simulink model "Power_MIL"  (R2024b)
settings: Solver=FixedStepAuto  StartTime=0.0  StopTime=50.0  FixedStep=0.01  RelTol=1e-3
undefined symbols (not defined in the file or in its folder): dcVoltage, Np, Ns, RegulatorLogicControl_12, RegulatorLogicControl_3, RegulatorLogicControl_5, sensor
libraries: nesl_utility x24, fl_lib x21, ee_lib x5, batt_lib x1, autolibdatasheetbattery x1, autolibdcdc x1
(part 2 of 2)

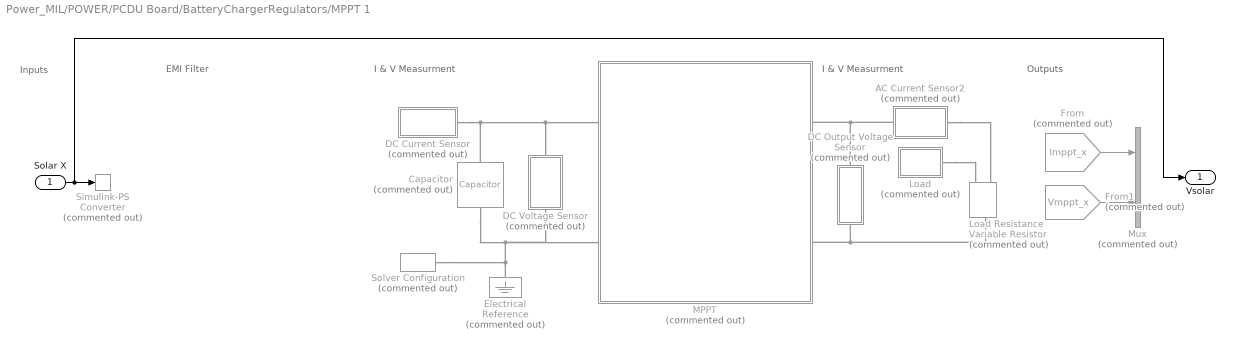
== system Power_MIL/POWER/PCDU Board/BatteryChargerRegulators/MPPT 1 ==
  note: Outputs
  note: Inputs
  note: I & V Measurment
  note: EMI Filter
  note: I & V Measurment
  Solar X : Inport
  AC Current Sensor2 : Subsystem  Commented=on
      mask Display: disp('i');
  Capacitor : fl_lib/Electrical/Electrical Elements/Capacitor  Commented=on  c=boost.inputCapacitor F  r=1e-6 Ohm  g=0 1/Ohm  i_specify=off  i_priority=None  i=0 A  i_nominal_specify=off  i_nominal_value=1  i_nominal_unit=A  v_specify=off  v_priority=None  v=solarPlant.startMPPTValue V  v_nominal_specify=off  v_nominal_value=1  v_nominal_unit=V  vc_specify=on  vc_priority=High  vc=solarPlant.startMPPTValue V  vc_nominal_specify=off  vc_nominal_value=1  vc_nominal_unit=V
  DC Current Sensor : Subsystem  Commented=on
      mask Display: disp('i')
  DC Output Voltage Sensor : Subsystem  Commented=on
      mask Display: disp('v')
  DC Voltage Sensor : Subsystem  Commented=on
      mask Display: disp('v');
  Electrical Reference : fl_lib/Electrical/Electrical Elements/Electrical Reference  Commented=on
  From : From  Commented=on  GotoTag=Imppt_x  TagVisibility=global
  From1 : From  Commented=on  GotoTag=Vmppt_x  TagVisibility=global
  Load : Subsystem  Commented=on
  Load Resistance : fl_lib/Electrical/Electrical Elements/Variable Resistor  Commented=on  Rmin=0 Ohm  thermalEnable=false  thermal_mass=1 J/K  i_specify=off  i_priority=None  i=5 A  i_nominal_specify=off  i_nominal_value=1  i_nominal_unit=A  v_specify=off  v_priority=None  v=0 V  v_nominal_specify=off  v_nominal_value=1  v_nominal_unit=V  T_specify=off  T_priority=None  T=300 K  T_nominal_specify=off  T_nominal_value=1  T_nominal_unit=K
  MPPT : Subsystem  Commented=on
  Mux : Mux  Commented=on  Inputs=2
  Simulink-PS Converter : nesl_utility/Simulink-PS Converter  Commented=on  PhysicalDomain=network_engine_domain  SubClassName=ps_input  LeftPortType=input  RightPortType=output  PseudoPeriodic=off  Frequencies=[]  NoiseDistribution=none  NoiseParameters=[]  Unit=1  AffineConversion=off  FilteringAndDerivatives=provide  SimscapeFilterOrder=1  InputFilterTimeConstant=0.001  UdotUserProvided=0
  Solver Configuration : nesl_utility/Solver Configuration  Commented=on  PhysicalDomain=network_engine_domain  SubClassName=solver  LeftPortType=input  RightPortType=generic  Tones=[]  Harmonics=[]  SimulateNoise=off  Profile=off  UseLocalSampling=off  EnableSwitchedLinearOptims=on  FrequencyDomain=off  UseCCode=off  RelTol=0.001  AbsTol=1e-06  MinStep=1e-09  ToWorkspace=off  RevertToSquareIcSolve=off  NumHomotopyIterations=100  PhasorMode=off  PhasorModeNumHarmonics=1  ConsistencySolver=NEWTON_FTOL  IndexReductionMethod=DerivativeReplacement  DoDC=off  ResidualTolerance=1e-9  ConsistencyTolSource=GLOBAL  ConsistencyAbsTol=0.001  ConsistencyRelTol=0.001  ConsistencyTolFactor=0.001  UseLocalSolver=off  LocalSolverChoice=NE_BACKWARD_EULER_ADVANCER  ResolveIndetEquations=on  FunctionEvalNumThread=1  LocalSolverSampleTime=1e-6  DoFixedCost=off  MaxNonlinIter=10  MaxModeIter=2  ComputeImpulses=off  ImpulseIterations=2  LinearAlgebra=auto  LinearAlgebraNumThread=0  EquationFormulation=NE_TIME_EF  DelaysMemoryBudget=1024  AutomaticFiltering=on  FilteringTimeConstant=0.001  PartitionStorageMethod=AS_NEEDED  PartitionMemoryBudget=1024  PartitionMethod=FAST  MultibodyUseLocalSolver=off  MultibodyLocalSolverChoice=ODE1  MultibodyLocalSolverSampleTime=0.001
  Vsolar : Outport
  wires:
  Solar X/1 -> Vsolar/1, Simulink-PS Converter/1
  From/1 -> Mux/1
  From1/1 -> Mux/2
  connections:
  Solver Configuration/RConn1 -- Capacitor/RConn1 -- DC Voltage Sensor/LConn1 -- MPPT/LConn2 -- Electrical Reference/LConn1
  DC Current Sensor/LConn1 -- DC Voltage Sensor/RConn1 -- MPPT/LConn1 -- Capacitor/LConn1
  Load Resistance/RConn1 -- MPPT/RConn2 -- DC Output Voltage Sensor/LConn1
  DC Output Voltage Sensor/RConn1 -- AC Current Sensor2/RConn1 -- MPPT/RConn1
  AC Current Sensor2/LConn1 -- Load Resistance/LConn2
  Load/RConn1 -- Load Resistance/LConn1

== system Power_MIL/POWER/PCDU Board/BatteryChargerRegulators/MPPT 2 ==
  Solar Y : Inport
  EMI Filters : Subsystem
  I & V Measurment : Subsystem
  I & V Measurment1 : Subsystem
  MPPT : Subsystem
  Vsolar : Outport
  wires:
  I & V Measurment1/1(V solar) -> Vsolar/1
  Solar Y/1 -> EMI Filters/1(In1)
  MPPT/1(Out1) -> I & V Measurment1/1(In1)
  I & V Measurment/1(V solar) -> MPPT/1(In1)
  EMI Filters/1(Solar X) -> I & V Measurment/1(Solar X)

== system Power_MIL/POWER/PCDU Board/BatteryChargerRegulators/MPPT 3 ==
  Solar Z : Inport
  EMI Filters : Subsystem
  I & V Measurment : Subsystem
  I & V Measurment1 : Subsystem
  MPPT : Subsystem
  Vsolar : Outport
  wires:
  I & V Measurment1/1(V solar) -> Vsolar/1
  Solar Z/1 -> EMI Filters/1(In1)
  MPPT/1(Out1) -> I & V Measurment1/1(In1)
  I & V Measurment/1(V solar) -> MPPT/1(In1)
  EMI Filters/1(Solar X) -> I & V Measurment/1(Solar X)

== system Power_MIL/POWER/PCDU Board/BatteryChargerRegulators/RBF ==
  In1 : Inport
  Constant : Constant  Value=[0 0]
  Manual Switch : ManualSwitch
  Hous Keeping1 : Outport
  wires:
  In1/1 -> Manual Switch/1
  Manual Switch/1 -> Hous Keeping1/1
  Constant/1 -> Manual Switch/2

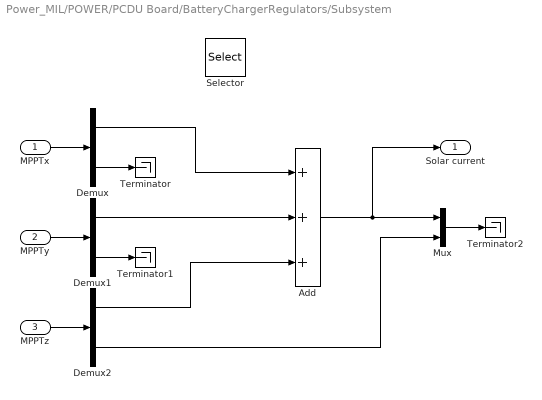
== system Power_MIL/POWER/PCDU Board/BatteryChargerRegulators/Subsystem ==
  MPPTx : Inport
  MPPTy : Inport  Port=2
  MPPTz : Inport  Port=3
  Add : Sum  Inputs=+++
  Demux : Demux  Outputs=2
  Demux1 : Demux  Outputs=2
  Demux2 : Demux  Outputs=2
  Mux : Mux  Inputs=2
  Selector : Selector  InputPortWidth=3  IndexOptions=Index vector (dialog)  Indices=[1 3]  OutputSizes=1
  Terminator : Terminator
  Terminator1 : Terminator
  Terminator2 : Terminator
  Solar current : Outport
  wires:
  MPPTx/1 -> Demux/1
  MPPTy/1 -> Demux1/1
  MPPTz/1 -> Demux2/1
  Demux1/1 -> Add/2
  Demux2/1 -> Add/3
  Add/1 -> Solar current/1, Mux/1
  Demux2/2 -> Mux/2
  Demux/1 -> Add/1
  Demux/2 -> Terminator/1
  Demux1/2 -> Terminator1/1
  Mux/1 -> Terminator2/1

== system Power_MIL/POWER/PCDU Board/BatteryChargerRegulators/current sense ==
  In1 : Inport
  Demux : Demux  Outputs=2
  Out1 : Outport
  tag scope: I_BCR=global
  wires:
  In1/1 -> Demux/1, Out1/1
  Demux/1 -> [I_BCR]

== system Power_MIL/POWER/PCDU Board/PowerConversionModules/Boost 12V ==
  In1 : Inport
  control_comm : Inport  Port=2
  Boost converter : Subsystem
  EMI Filter in : Subsystem
  EMI Filter out : Subsystem
  CV : Outport
  LogicControl_Out : Outport  Port=2
  wires:
  EMI Filter in/1(Out1) -> Boost converter/1(CV_in)
  Boost converter/1(CV_out) -> EMI Filter out/1(In1)
  In1/1 -> EMI Filter in/1(In1)
  EMI Filter out/1(Out1) -> CV/1
  control_comm/1 -> Boost converter/2(LogicControl_in)
  Boost converter/2(LogicControl_out) -> LogicControl_Out/1

== system Power_MIL/POWER/PCDU Board/PowerConversionModules/Boost_12V ==
  BatteryVoltage : Inport
  Gain : Gain  Gain=12/6.5
  12V : Outport
  wires:
  BatteryVoltage/1 -> Gain/1
  Gain/1 -> 12V/1

== system Power_MIL/POWER/PCDU Board/PowerConversionModules/Boost_3.3V ==
  BatteryVoltage : Inport
  Gain : Gain  Gain=3.3/6.5
  12V : Outport
  wires:
  BatteryVoltage/1 -> Gain/1
  Gain/1 -> 12V/1

== system Power_MIL/POWER/PCDU Board/PowerConversionModules/Boost_5V ==
  BatteryVoltage : Inport
  Gain : Gain  Gain=5/6.5
  12V : Outport
  wires:
  Gain/1 -> 12V/1
  BatteryVoltage/1 -> Gain/1

== system Power_MIL/POWER/PCDU Board/PowerConversionModules/Buck 3.3_1 ==
  Inport : Inport
  control_comm : Inport  Port=2
  Boost converter : Subsystem
  EMI Filter in : Subsystem
  EMI Filter out : Subsystem
  v_3.3_1 : Outport
  LogicControl_Out : Outport  Port=2
  wires:
  EMI Filter in/1(CV_in) -> Boost converter/1(CV_in)
  Boost converter/1(CV_out) -> EMI Filter out/1(CV_out)
  Inport/1 -> EMI Filter in/1(In1)
  EMI Filter out/1(Out1) -> v_3.3_1/1
  control_comm/1 -> Boost converter/2(LogicControl_in)
  Boost converter/2(LogicControl_out) -> LogicControl_Out/1

== system Power_MIL/POWER/PCDU Board/PowerConversionModules/Buck 3.3_2 ==
  In1 : Inport
  control_comm : Inport  Port=2
  Boost converter : Subsystem
  EMI Filter in : Subsystem
  EMI Filter out : Subsystem
  Output : Outport
  LogicControl_Out : Outport  Port=2
  wires:
  In1/1 -> EMI Filter in/1(In1)
  EMI Filter out/1(Output) -> Output/1
  EMI Filter in/1(CV_in) -> Boost converter/1(CV_in)
  Boost converter/1(CV_out) -> EMI Filter out/1(CV_out)
  control_comm/1 -> Boost converter/2(LogicControl_in)
  Boost converter/2(LogicControl_out) -> LogicControl_Out/1

== system Power_MIL/POWER/PCDU Board/PowerConversionModules/Buck 5 ==
  In1 : Inport
  control_comm : Inport  Port=2
  Boost converter : Subsystem
  EMI Filter in : Subsystem
  EMI Filter out : Subsystem
  V_5 : Outport
  LogicControl_Out : Outport  Port=2
  wires:
  EMI Filter in/1(Out1) -> Boost converter/1(CV_in)
  Boost converter/1(CV_out) -> EMI Filter out/1(In1)
  In1/1 -> EMI Filter in/1(In1)
  EMI Filter out/1(Out1) -> V_5/1
  control_comm/1 -> Boost converter/2(LogicControl_in)
  Boost converter/2(LogicControl_out) -> LogicControl_Out/1

== system Power_MIL/POWER/PCDU Board/PowerConversionModules/I and V Measurment ==
  In1 : Inport
  V_12 : Outport
  wires:
  In1/1 -> V_12/1

== system Power_MIL/POWER/PCDU Board/PowerConversionModules/LCL in 12 ==
  In1 : Inport
  Out1 : Outport
  wires:
  In1/1 -> Out1/1

== system Power_MIL/POWER/PCDU Board/PowerDistributionModules/LCL out 1 ==
  V_12 : Inport
  Demux : Demux  Outputs=2
  Voltage_5 : Outport
  wires:
  V_12/1 -> Demux/1
  Demux/2 -> Voltage_5/1

== system Power_MIL/POWER/PCDU Board/PowerDistributionModules/LCL out 12 ==
  V_12 : Inport
  Demux : Demux  Outputs=2
  Voltage_12 : Outport
  wires:
  V_12/1 -> Demux/1

== system Power_MIL/POWER/PCDU Board/PowerDistributionModules/LCL out 2 ==
  V_3.3_1 : Inport
  V_3.3_2 : Inport  Port=2
  Demux : Demux  Outputs=2
  Scope : Scope
  Voltage_3.3 : Outport
  wires:
  V_3.3_2/1 -> Scope/1
  V_3.3_1/1 -> Demux/1
  Demux/2 -> Voltage_3.3/1

== system Power_MIL/POWER/PCDU Board/PowerDistributionModules/current sense2 ==
  CV_in : Inport
  Demux : Demux  Outputs=2
  Mux : Mux  Inputs=2
  CV_Converter : Outport
  I_Converter : Outport  Port=2
  wires:
  CV_in/1 -> Demux/1
  Demux/1 -> I_Converter/1, Mux/1
  Demux/2 -> Mux/2
  Mux/1 -> CV_Converter/1

== system Power_MIL/POWER/Solar Panels/Solar Panel +X/Solar Panel1 ==
  Current-Controlled Current Source : fl_lib/Electrical/Electrical Sources/Current-Controlled Current Source  K=-1  i1_specify=off  i1_priority=None  i1=0 A  i1_nominal_specify=off  i1_nominal_value=1  i1_nominal_unit=A  i2_specify=off  i2_priority=None  i2=0 A  i2_nominal_specify=off  i2_nominal_value=1  i2_nominal_unit=A
      settings: InternalSimscapePortConfiguration="{\"Bottom\":[],\"Left\":[{\"id\":\"p1\",\"label\":\"+\",\"type\":\"foundation.electrical.electrical\"},{\"id\":\"head\",\"label\":\"\",\"type\":\"foundation.electrical.electrical\"}],\"Right\":[{\"id\":\"n1\",\"label\":\"-\",\"type\":\"foundation.electrical.electrical\"},{\"id\":\"tail\",\"label\":\"\",\"type\":\"foundation.electrical.electrical\"}],\"Top\":[]}"
  Solar Cell : ee_lib/Sources/Solar Cell  PartSpecification="{\"DatasetId\":\"AzurSpace|3C44_30sqmm|simscape.electrical.solarCell\",\"DisplayName\":\"AzurSpace:3C44_30sqmm\"}"  prm=3  Isc=1.19 % Datasheet derived A  Voc=3.08 % Datasheet derived V  Is=2.73592960844769e-35 % Datasheet derived A  Is2=1.16779785679844e-37 % Datasheet derived A  Iph=1.19000472592367 % Datasheet derived A  Ir0=250000 % Datasheet derived W/m^2  ec=1.50303550965723 % Datasheet derived  N2=1.59525933684062 % Datasheet derived  Rs=0.104281524604326 % Datasheet derived Ohm  Rp=26248.1045129446 % Datasheet derived Ohm  N_series=1 % Datasheet derived  N_parallel=1 % Datasheet derived  TIPH1=0.000799987520460482 % Datasheet derived 1/K  EG=1.441 % Datasheet derived eV  TXIS1=92.8777524632801 % Datasheet derived  TXIS2=227.92622072394 % Datasheet derived  TRS1=0.0216421647602992 % Datasheet derived  TRP1=0 % Parameter not set  Tmeas=25 % Datasheet derived degC  TFIXED=25 % Datasheet derived degC  thermal_mass=100 % Parameter not set J/K  initial_temperature=25 degC
      settings: AttributesFormatString=AzurSpace:3C44_30sqmm
  Ir : PMIOPort  Side=Left
  + : PMIOPort  Port=2  Side=Right
  - : PMIOPort  Port=3  Side=Right
  connections:
  +/RConn1 -- Current-Controlled Current Source/RConn2 -- Current-Controlled Current Source/RConn1
  Current-Controlled Current Source/LConn1 -- Solar Cell/LConn2
  Ir/RConn1 -- Solar Cell/LConn1
  Solar Cell/RConn1 -- -/RConn1 -- Current-Controlled Current Source/LConn2

== system Power_MIL/POWER/Solar Panels/Solar Panel +Y/Solar Panel1 ==
  Current-Controlled Current Source : fl_lib/Electrical/Electrical Sources/Current-Controlled Current Source  K=-1  i1_specify=off  i1_priority=None  i1=0 A  i1_nominal_specify=off  i1_nominal_value=1  i1_nominal_unit=A  i2_specify=off  i2_priority=None  i2=0 A  i2_nominal_specify=off  i2_nominal_value=1  i2_nominal_unit=A
      settings: InternalSimscapePortConfiguration="{\"Bottom\":[],\"Left\":[{\"id\":\"p1\",\"label\":\"+\",\"type\":\"foundation.electrical.electrical\"},{\"id\":\"head\",\"label\":\"\",\"type\":\"foundation.electrical.electrical\"}],\"Right\":[{\"id\":\"n1\",\"label\":\"-\",\"type\":\"foundation.electrical.electrical\"},{\"id\":\"tail\",\"label\":\"\",\"type\":\"foundation.electrical.electrical\"}],\"Top\":[]}"
  Solar Cell : ee_lib/Sources/Solar Cell  PartSpecification="{\"DatasetId\":\"AzurSpace|3C44_30sqmm|simscape.electrical.solarCell\",\"DisplayName\":\"AzurSpace:3C44_30sqmm\"}"  prm=3  Isc=1.19 % Datasheet derived A  Voc=3.08 % Datasheet derived V  Is=2.73592960844769e-35 % Datasheet derived A  Is2=1.16779785679844e-37 % Datasheet derived A  Iph=1.19000472592367 % Datasheet derived A  Ir0=250000 % Datasheet derived W/m^2  ec=1.50303550965723 % Datasheet derived  N2=1.59525933684062 % Datasheet derived  Rs=0.104281524604326 % Datasheet derived Ohm  Rp=26248.1045129446 % Datasheet derived Ohm  N_series=1 % Datasheet derived  N_parallel=1 % Datasheet derived  TIPH1=0.000799987520460482 % Datasheet derived 1/K  EG=1.441 % Datasheet derived eV  TXIS1=92.8777524632801 % Datasheet derived  TXIS2=227.92622072394 % Datasheet derived  TRS1=0.0216421647602992 % Datasheet derived  TRP1=0 % Parameter not set  Tmeas=25 % Datasheet derived degC  TFIXED=25 % Datasheet derived degC  thermal_mass=100 % Parameter not set J/K  initial_temperature=25 degC
      settings: AttributesFormatString=AzurSpace:3C44_30sqmm
  Ir : PMIOPort  Side=Left
  + : PMIOPort  Port=2  Side=Right
  - : PMIOPort  Port=3  Side=Right
  connections:
  +/RConn1 -- Current-Controlled Current Source/RConn2 -- Current-Controlled Current Source/RConn1
  Current-Controlled Current Source/LConn1 -- Solar Cell/LConn2
  Ir/RConn1 -- Solar Cell/LConn1
  Solar Cell/RConn1 -- -/RConn1 -- Current-Controlled Current Source/LConn2

== system Power_MIL/POWER/Solar Panels/Solar Panel -X/Solar Panel2 ==
  Current-Controlled Current Source : fl_lib/Electrical/Electrical Sources/Current-Controlled Current Source  K=-1  i1_specify=off  i1_priority=None  i1=0 A  i1_nominal_specify=off  i1_nominal_value=1  i1_nominal_unit=A  i2_specify=off  i2_priority=None  i2=0 A  i2_nominal_specify=off  i2_nominal_value=1  i2_nominal_unit=A
      settings: InternalSimscapePortConfiguration="{\"Bottom\":[],\"Left\":[{\"id\":\"p1\",\"label\":\"+\",\"type\":\"foundation.electrical.electrical\"},{\"id\":\"head\",\"label\":\"\",\"type\":\"foundation.electrical.electrical\"}],\"Right\":[{\"id\":\"n1\",\"label\":\"-\",\"type\":\"foundation.electrical.electrical\"},{\"id\":\"tail\",\"label\":\"\",\"type\":\"foundation.electrical.electrical\"}],\"Top\":[]}"
  Solar Cell : ee_lib/Sources/Solar Cell  PartSpecification="{\"DatasetId\":\"AzurSpace|3C44_30sqmm|simscape.electrical.solarCell\",\"DisplayName\":\"AzurSpace:3C44_30sqmm\"}"  prm=3  Isc=1.19 % Datasheet derived A  Voc=3.08 % Datasheet derived V  Is=2.73592960844769e-35 % Datasheet derived A  Is2=1.16779785679844e-37 % Datasheet derived A  Iph=1.19000472592367 % Datasheet derived A  Ir0=250000 % Datasheet derived W/m^2  ec=1.50303550965723 % Datasheet derived  N2=1.59525933684062 % Datasheet derived  Rs=0.104281524604326 % Datasheet derived Ohm  Rp=26248.1045129446 % Datasheet derived Ohm  N_series=1 % Datasheet derived  N_parallel=1 % Datasheet derived  TIPH1=0.000799987520460482 % Datasheet derived 1/K  EG=1.441 % Datasheet derived eV  TXIS1=92.8777524632801 % Datasheet derived  TXIS2=227.92622072394 % Datasheet derived  TRS1=0.0216421647602992 % Datasheet derived  TRP1=0 % Parameter not set  Tmeas=25 % Datasheet derived degC  TFIXED=25 % Datasheet derived degC  thermal_mass=100 % Parameter not set J/K  initial_temperature=25 degC
      settings: AttributesFormatString=AzurSpace:3C44_30sqmm
  Ir : PMIOPort  Side=Left
  + : PMIOPort  Port=2  Side=Right
  - : PMIOPort  Port=3  Side=Right
  connections:
  +/RConn1 -- Current-Controlled Current Source/RConn2 -- Current-Controlled Current Source/RConn1
  Current-Controlled Current Source/LConn1 -- Solar Cell/LConn2
  Ir/RConn1 -- Solar Cell/LConn1
  Solar Cell/RConn1 -- -/RConn1 -- Current-Controlled Current Source/LConn2

== system Power_MIL/POWER/Solar Panels/Solar Panel -Y/Solar Panel1 ==
  Current-Controlled Current Source : fl_lib/Electrical/Electrical Sources/Current-Controlled Current Source  K=-1  i1_specify=off  i1_priority=None  i1=0 A  i1_nominal_specify=off  i1_nominal_value=1  i1_nominal_unit=A  i2_specify=off  i2_priority=None  i2=0 A  i2_nominal_specify=off  i2_nominal_value=1  i2_nominal_unit=A
      settings: InternalSimscapePortConfiguration="{\"Bottom\":[],\"Left\":[{\"id\":\"p1\",\"label\":\"+\",\"type\":\"foundation.electrical.electrical\"},{\"id\":\"head\",\"label\":\"\",\"type\":\"foundation.electrical.electrical\"}],\"Right\":[{\"id\":\"n1\",\"label\":\"-\",\"type\":\"foundation.electrical.electrical\"},{\"id\":\"tail\",\"label\":\"\",\"type\":\"foundation.electrical.electrical\"}],\"Top\":[]}"
  Solar Cell : ee_lib/Sources/Solar Cell  PartSpecification="{\"DatasetId\":\"AzurSpace|3C44_30sqmm|simscape.electrical.solarCell\",\"DisplayName\":\"AzurSpace:3C44_30sqmm\"}"  prm=3  Isc=1.19 % Datasheet derived A  Voc=3.08 % Datasheet derived V  Is=2.73592960844769e-35 % Datasheet derived A  Is2=1.16779785679844e-37 % Datasheet derived A  Iph=1.19000472592367 % Datasheet derived A  Ir0=250000 % Datasheet derived W/m^2  ec=1.50303550965723 % Datasheet derived  N2=1.59525933684062 % Datasheet derived  Rs=0.104281524604326 % Datasheet derived Ohm  Rp=26248.1045129446 % Datasheet derived Ohm  N_series=1 % Datasheet derived  N_parallel=1 % Datasheet derived  TIPH1=0.000799987520460482 % Datasheet derived 1/K  EG=1.441 % Datasheet derived eV  TXIS1=92.8777524632801 % Datasheet derived  TXIS2=227.92622072394 % Datasheet derived  TRS1=0.0216421647602992 % Datasheet derived  TRP1=0 % Parameter not set  Tmeas=25 % Datasheet derived degC  TFIXED=25 % Datasheet derived degC  thermal_mass=100 % Parameter not set J/K  initial_temperature=25 degC
      settings: AttributesFormatString=AzurSpace:3C44_30sqmm
  Solver Configuration : nesl_utility/Solver Configuration  PhysicalDomain=network_engine_domain  SubClassName=solver  LeftPortType=input  RightPortType=generic  Tones=[]  Harmonics=[]  SimulateNoise=off  Profile=off  UseLocalSampling=off  EnableSwitchedLinearOptims=on  FrequencyDomain=off  UseCCode=off  RelTol=0.001  AbsTol=0.001  MinStep=1e-09  ToWorkspace=off  RevertToSquareIcSolve=off  NumHomotopyIterations=100  PhasorMode=off  PhasorModeNumHarmonics=1  ConsistencySolver=NEWTON_XTOL_AFTER_FTOL  IndexReductionMethod=DerivativeReplacement  DoDC=off  ResidualTolerance=1e-09  ConsistencyTolSource=GLOBAL  ConsistencyAbsTol=0.001  ConsistencyRelTol=0.001  ConsistencyTolFactor=0.001  UseLocalSolver=off  LocalSolverChoice=NE_BACKWARD_EULER_ADVANCER  ResolveIndetEquations=on  FunctionEvalNumThread=1  LocalSolverSampleTime=0.001  DoFixedCost=off  MaxNonlinIter=3  MaxModeIter=2  ComputeImpulses=off  ImpulseIterations=2  LinearAlgebra=auto  LinearAlgebraNumThread=0  EquationFormulation=NE_TIME_EF  DelaysMemoryBudget=1024  AutomaticFiltering=on  FilteringTimeConstant=0.001  PartitionStorageMethod=AS_NEEDED  PartitionMemoryBudget=1024  PartitionMethod=ROBUST  MultibodyUseLocalSolver=off  MultibodyLocalSolverChoice=ODE1  MultibodyLocalSolverSampleTime=0.001
  Ir : PMIOPort  Side=Left
  + : PMIOPort  Port=2  Side=Right
  - : PMIOPort  Port=3  Side=Right
  connections:
  +/RConn1 -- Current-Controlled Current Source/RConn2 -- Current-Controlled Current Source/RConn1
  Current-Controlled Current Source/LConn1 -- Solar Cell/LConn2
  Ir/RConn1 -- Solver Configuration/RConn1 -- Solar Cell/LConn1
  Solar Cell/RConn1 -- -/RConn1 -- Current-Controlled Current Source/LConn2

== system Power_MIL/POWER/Solar Panels/Solar Panel Z/Solar Panel1 ==
  Current-Controlled Current Source : fl_lib/Electrical/Electrical Sources/Current-Controlled Current Source  K=-1  i1_specify=off  i1_priority=None  i1=0 A  i1_nominal_specify=off  i1_nominal_value=1  i1_nominal_unit=A  i2_specify=off  i2_priority=None  i2=0 A  i2_nominal_specify=off  i2_nominal_value=1  i2_nominal_unit=A
      settings: InternalSimscapePortConfiguration="{\"Bottom\":[],\"Left\":[{\"id\":\"p1\",\"label\":\"+\",\"type\":\"foundation.electrical.electrical\"},{\"id\":\"head\",\"label\":\"\",\"type\":\"foundation.electrical.electrical\"}],\"Right\":[{\"id\":\"n1\",\"label\":\"-\",\"type\":\"foundation.electrical.electrical\"},{\"id\":\"tail\",\"label\":\"\",\"type\":\"foundation.electrical.electrical\"}],\"Top\":[]}"
  Solar Cell : ee_lib/Sources/Solar Cell  PartSpecification="{\"DatasetId\":\"AzurSpace|3C44_30sqmm|simscape.electrical.solarCell\",\"DisplayName\":\"AzurSpace:3C44_30sqmm\"}"  prm=3  Isc=1.19 % Datasheet derived A  Voc=3.08 % Datasheet derived V  Is=2.73592960844769e-35 % Datasheet derived A  Is2=1.16779785679844e-37 % Datasheet derived A  Iph=1.19000472592367 % Datasheet derived A  Ir0=250000 % Datasheet derived W/m^2  ec=1.50303550965723 % Datasheet derived  N2=1.59525933684062 % Datasheet derived  Rs=0.104281524604326 % Datasheet derived Ohm  Rp=26248.1045129446 % Datasheet derived Ohm  N_series=1 % Datasheet derived  N_parallel=1 % Datasheet derived  TIPH1=0.000799987520460482 % Datasheet derived 1/K  EG=1.441 % Datasheet derived eV  TXIS1=92.8777524632801 % Datasheet derived  TXIS2=227.92622072394 % Datasheet derived  TRS1=0.0216421647602992 % Datasheet derived  TRP1=0 % Parameter not set  Tmeas=25 % Datasheet derived degC  TFIXED=25 % Datasheet derived degC  thermal_mass=100 % Parameter not set J/K  initial_temperature=25 degC
      settings: AttributesFormatString=AzurSpace:3C44_30sqmm
  Ir : PMIOPort  Side=Left
  + : PMIOPort  Port=2  Side=Right
  - : PMIOPort  Port=3  Side=Right
  connections:
  +/RConn1 -- Current-Controlled Current Source/RConn2 -- Current-Controlled Current Source/RConn1
  Current-Controlled Current Source/LConn1 -- Solar Cell/LConn2
  Ir/RConn1 -- Solar Cell/LConn1
  Solar Cell/RConn1 -- -/RConn1 -- Current-Controlled Current Source/LConn2

== system Power_MIL/POWER/PCDU Board/BatteryChargerRegulators/MPPT 1/AC Current Sensor2 ==
  Current Sensor : fl_lib/Electrical/Electrical Sensors/Current Sensor
  PS-Simulink Converter : nesl_utility/PS-Simulink Converter  PhysicalDomain=network_engine_domain  SubClassName=ps_output  LeftPortType=input  RightPortType=output  PseudoPeriodic=off  Frequencies=[]  VectorFormat=1-D array  Unit=1  AffineConversion=off
  Sensor dynamics : TransferFcn  Numerator=1  Denominator=[1/sensor.samplingFreq 1]
  - : PMIOPort  Side=Left
  + : PMIOPort  Port=2  Side=Right
  tag scope: Imppt_x=global
  wires:
  Sensor dynamics/1 -> [Imppt_x]
  PS-Simulink Converter/1 -> Sensor dynamics/1
  connections:
  Current Sensor/RConn2 -- -/RConn1
  +/RConn1 -- Current Sensor/LConn1
  Current Sensor/RConn1 -- PS-Simulink Converter/LConn1

== system Power_MIL/POWER/PCDU Board/BatteryChargerRegulators/MPPT 1/DC Current Sensor ==
  Current Sensor : fl_lib/Electrical/Electrical Sensors/Current Sensor
      settings: LogSimulationData=on
  PS-Simulink Converter : nesl_utility/PS-Simulink Converter  PhysicalDomain=network_engine_domain  SubClassName=ps_output  LeftPortType=input  RightPortType=output  PseudoPeriodic=off  Frequencies=[]  VectorFormat=1-D array  Unit=1  AffineConversion=off
  Sensor dynamics : TransferFcn  Numerator=1  Denominator=[1/sensor.samplingFreq 1]
  - : PMIOPort  Side=Left
  + : PMIOPort  Port=2  Side=Right
  tag scope: Icell_x=global
  wires:
  Sensor dynamics/1 -> [Icell_x]
  PS-Simulink Converter/1 -> Sensor dynamics/1
  connections:
  Current Sensor/RConn1 -- PS-Simulink Converter/LConn1
  +/RConn1 -- Current Sensor/LConn1
  Current Sensor/RConn2 -- -/RConn1

== system Power_MIL/POWER/PCDU Board/BatteryChargerRegulators/MPPT 1/DC Output Voltage Sensor ==
  PS-Simulink Converter : nesl_utility/PS-Simulink Converter  PhysicalDomain=network_engine_domain  SubClassName=ps_output  LeftPortType=input  RightPortType=output  PseudoPeriodic=off  Frequencies=[]  VectorFormat=1-D array  Unit=1  AffineConversion=off
  Sensor dynamics : TransferFcn  Numerator=1  Denominator=[1/sensor.samplingFreq 1]
  Voltage Sensor : fl_lib/Electrical/Electrical Sensors/Voltage Sensor
  - : PMIOPort  Side=Left
  + : PMIOPort  Port=2  Side=Right
  tag scope: Vmppt_x=global
  wires:
  Sensor dynamics/1 -> [Vmppt_x]
  PS-Simulink Converter/1 -> Sensor dynamics/1
  connections:
  Voltage Sensor/LConn1 -- +/RConn1
  Voltage Sensor/RConn1 -- PS-Simulink Converter/LConn1
  Voltage Sensor/RConn2 -- -/RConn1

== system Power_MIL/POWER/PCDU Board/BatteryChargerRegulators/MPPT 1/DC Voltage Sensor ==
  PS-Simulink Converter : nesl_utility/PS-Simulink Converter  PhysicalDomain=network_engine_domain  SubClassName=ps_output  LeftPortType=input  RightPortType=output  PseudoPeriodic=off  Frequencies=[]  VectorFormat=1-D array  Unit=1  AffineConversion=off
  Sensor dynamics : TransferFcn  Numerator=1  Denominator=[1/sensor.samplingFreq 1]
  Voltage Sensor : fl_lib/Electrical/Electrical Sensors/Voltage Sensor
      settings: LogSimulationData=on
  - : PMIOPort  Side=Left
  + : PMIOPort  Port=2  Side=Right
  tag scope: Vcell_x=global
  wires:
  Sensor dynamics/1 -> [Vcell_x]
  PS-Simulink Converter/1 -> Sensor dynamics/1
  connections:
  Voltage Sensor/RConn2 -- -/RConn1
  Voltage Sensor/RConn1 -- PS-Simulink Converter/LConn1
  Voltage Sensor/LConn1 -- +/RConn1

== system Power_MIL/POWER/PCDU Board/BatteryChargerRegulators/MPPT 1/Load ==
  " " : Constant
  " (Average DC Voltage)^2" : Constant  Value=dcVoltage.avgDCVoltage*dcVoltage.avgDCVoltage
  " 1" : Constant  Value=1.5
  Load Power (kW) : Gain  Gain=1.688857025146485
  Simulink-PS Converter1 : nesl_utility/Simulink-PS Converter  PhysicalDomain=network_engine_domain  SubClassName=ps_input  LeftPortType=input  RightPortType=output  PseudoPeriodic=off  Frequencies=[]  NoiseDistribution=none  NoiseParameters=[]  Unit=1  AffineConversion=off  FilteringAndDerivatives=provide  SimscapeFilterOrder=1  InputFilterTimeConstant=0.001  UdotUserProvided=0
  Switch : Switch  Criteria=u2 > Threshold  SaturateOnIntegerOverflow=off  InputSameDT=off
  V^2/P : Product  Inputs=*/
  kW2W : Gain  Gain=1000
  R : PMIOPort  Side=Right
  wires:
  kW2W/1 -> V^2/P/2
  Switch/1 -> kW2W/1
  V^2/P/1 -> Simulink-PS Converter1/1
  " (Average DC Voltage)^2"/1 -> V^2/P/1
  " 1"/1 -> Switch/3
  Load Power (kW)/1 -> Switch/2, Switch/1
  " "/1 -> Load Power (kW)/1
  connections:
  Simulink-PS Converter1/RConn1 -- R/RConn1

== system Power_MIL/POWER/PCDU Board/BatteryChargerRegulators/MPPT 1/MPPT ==
  Bus Selector : BusSelector  OutputSignals=signal1
  SEPIC converter : Subsystem
  Switch1 : Switch  SaturateOnIntegerOverflow=off  InputSameDT=off
  in + : PMIOPort  Side=Left
  in - : PMIOPort  Port=2  Side=Left
  out + : PMIOPort  Port=3  Side=Right
  out - : PMIOPort  Port=4  Side=Right
  wires:
  [control_comm] -> Bus Selector/1

== system Power_MIL/POWER/PCDU Board/BatteryChargerRegulators/MPPT 2/EMI Filters ==
  In1 : Inport
  Solar X : Outport
  wires:
  In1/1 -> Solar X/1

== system Power_MIL/POWER/PCDU Board/BatteryChargerRegulators/MPPT 2/I & V Measurment ==
  Solar X : Inport
  V solar : Outport
  wires:
  Solar X/1 -> V solar/1

== system Power_MIL/POWER/PCDU Board/BatteryChargerRegulators/MPPT 2/I & V Measurment1 ==
  In1 : Inport
  V solar : Outport
  wires:
  In1/1 -> V solar/1

== system Power_MIL/POWER/PCDU Board/BatteryChargerRegulators/MPPT 2/MPPT ==
  In1 : Inport
  SEPIC converter : Subsystem
  Out1 : Outport
  wires:
  In1/1 -> SEPIC converter/1(In1)
  SEPIC converter/1(Out1) -> Out1/1

== system Power_MIL/POWER/PCDU Board/BatteryChargerRegulators/MPPT 3/EMI Filters ==
  In1 : Inport
  Solar X : Outport
  wires:
  In1/1 -> Solar X/1

== system Power_MIL/POWER/PCDU Board/BatteryChargerRegulators/MPPT 3/I & V Measurment ==
  Solar X : Inport
  V solar : Outport
  wires:
  Solar X/1 -> V solar/1

== system Power_MIL/POWER/PCDU Board/BatteryChargerRegulators/MPPT 3/I & V Measurment1 ==
  In1 : Inport
  V solar : Outport
  wires:
  In1/1 -> V solar/1

== system Power_MIL/POWER/PCDU Board/BatteryChargerRegulators/MPPT 3/MPPT ==
  In1 : Inport
  SEPIC converter : Subsystem
  Out1 : Outport
  wires:
  In1/1 -> SEPIC converter/1(In1)
  SEPIC converter/1(Out1) -> Out1/1

== system Power_MIL/POWER/PCDU Board/PowerConversionModules/Boost 12V/Boost converter ==
  CV_in : Inport
  LogicControl_in : Inport  Port=2
  CV_out : Outport
  LogicControl_out : Outport  Port=2
  wires:
  CV_in/1 -> CV_out/1
  LogicControl_in/1 -> LogicControl_out/1

== system Power_MIL/POWER/PCDU Board/PowerConversionModules/Boost 12V/EMI Filter in ==
  In1 : Inport
  Out1 : Outport
  wires:
  In1/1 -> Out1/1

== system Power_MIL/POWER/PCDU Board/PowerConversionModules/Boost 12V/EMI Filter out ==
  In1 : Inport
  Out1 : Outport
  wires:
  In1/1 -> Out1/1

== system Power_MIL/POWER/PCDU Board/PowerConversionModules/Buck 3.3_1/Boost converter ==
  CV_in : Inport
  LogicControl_in : Inport  Port=2
  CV_out : Outport
  LogicControl_out : Outport  Port=2
  wires:
  CV_in/1 -> CV_out/1
  LogicControl_in/1 -> LogicControl_out/1

== system Power_MIL/POWER/PCDU Board/PowerConversionModules/Buck 3.3_1/EMI Filter in ==
  In1 : Inport
  CV_in : Outport
  wires:
  In1/1 -> CV_in/1

== system Power_MIL/POWER/PCDU Board/PowerConversionModules/Buck 3.3_1/EMI Filter out ==
  CV_out : Inport
  Out1 : Outport
  wires:
  CV_out/1 -> Out1/1

== system Power_MIL/POWER/PCDU Board/PowerConversionModules/Buck 3.3_2/Boost converter ==
  CV_in : Inport
  LogicControl_in : Inport  Port=2
  CV_out : Outport
  LogicControl_out : Outport  Port=2
  wires:
  CV_in/1 -> CV_out/1
  LogicControl_in/1 -> LogicControl_out/1

== system Power_MIL/POWER/PCDU Board/PowerConversionModules/Buck 3.3_2/EMI Filter in ==
  In1 : Inport
  CV_in : Outport
  wires:
  In1/1 -> CV_in/1

== system Power_MIL/POWER/PCDU Board/PowerConversionModules/Buck 3.3_2/EMI Filter out ==
  CV_out : Inport
  Output : Outport
  wires:
  CV_out/1 -> Output/1

== system Power_MIL/POWER/PCDU Board/PowerConversionModules/Buck 5/Boost converter ==
  CV_in : Inport
  LogicControl_in : Inport  Port=2
  CV_out : Outport
  LogicControl_out : Outport  Port=2
  wires:
  CV_in/1 -> CV_out/1
  LogicControl_in/1 -> LogicControl_out/1

== system Power_MIL/POWER/PCDU Board/PowerConversionModules/Buck 5/EMI Filter in ==
  In1 : Inport
  Out1 : Outport
  wires:
  In1/1 -> Out1/1

== system Power_MIL/POWER/PCDU Board/PowerConversionModules/Buck 5/EMI Filter out ==
  In1 : Inport
  Out1 : Outport
  wires:
  In1/1 -> Out1/1

== system Power_MIL/POWER/PCDU Board/BatteryChargerRegulators/MPPT 1/MPPT/SEPIC converter ==
  In1 : Inport
  Out1 : Outport
  wires:
  In1/1 -> Out1/1

== system Power_MIL/POWER/PCDU Board/BatteryChargerRegulators/MPPT 2/MPPT/SEPIC converter ==
  In1 : Inport
  Out1 : Outport
  wires:
  In1/1 -> Out1/1

== system Power_MIL/POWER/PCDU Board/BatteryChargerRegulators/MPPT 3/MPPT/SEPIC converter ==
  In1 : Inport
  Out1 : Outport
  wires:
  In1/1 -> Out1/1

== matlab function Power_MIL/POWER/Battery/Balancing algorithm/Algorithm/Cell Balancing Algorithm ==
  data: I input; minSOC input; indx_minSOC input; deltaSOC output; maxSOC input; indx_maxSOC input; SW output; minT input; maxT input; Ns parameter; Np parameter
function [deltaSOC,SW] = cellBalancing(I,minSOC,indx_minSOC,maxSOC,indx_maxSOC,minT,maxT, Ns, Np)
%% User input
lim_percentSOC=0.05;
%% Cell balancing logic
SW=zeros(1,Ns);
deltaSOC=(maxSOC-minSOC)*100;
% Start cell balancing only if battery is not being used (I==0)
if deltaSOC > lim_percentSOC && I == 0
    if Np==1
        indx_minSOC_SWnum=indx_minSOC;
    else
        indx_minSOC_SWnum=(indx_minSOC-mod(indx_minSOC,Np))/Np+1;
    end
    for i=1:Ns
        if i==indx_minSOC_SWnum
            SW(1,i)=0;
        else
            SW(1,i)=1;
        end
    end
end

end

== matlab function Power_MIL/EPS software/MATLAB Function1 ==
  data: Power_consumption input; TotalCurrent output
function TotalCurrent = fcn(Power_consumption)

TotalCurrent = 0;

for i = 1:length(Power_consumption)/2

    TotalCurrent = TotalCurrent + Power_consumption(2*(i),1);
end
1
% TotalCurrent = sum(Power_consumption(:,2));

end

== matlab function Power_MIL/POWER/Battery/Balancing algorithm/SOC & T min//max/SOC ==
  data: SOC input; minSOC output; minSOCindx output; maxSOC output; maxSOCindx output
function [minSOC,minSOCindx,maxSOC,maxSOCindx] = fcn(SOC)
maxSOC=max(SOC);
minSOC=min(SOC);
minSOCidx=find(SOC==minSOC);
maxSOCidx=find(SOC==maxSOC);
minSOCindx=minSOCidx(1);
maxSOCindx=maxSOCidx(1);
